simulink model "EkalmanF_ac_sim"  (R2025b)
settings: Solver=VariableStepAuto  StartTime=0.0  StopTime=StopTime  RelTol=1e-3
values from neighbouring files (symbols this model uses):
  B = [0.5*dt^2 0 ... (first row only)    [Extended_Kalman_Filter.m]    (also in Kalman_filter.m; kalman_ac.m = fi(B, true, 32, 20))
  C = fi(C, true, 32, 20)    [kalman_ac.m]
  dt = 0.2    [Extended_Kalman_Filter.m]    (also in Kalman_filter.m; UKF.m; kalman_ac.m = 0.02)
  H = [1 0 0 0 ... (first row only)    [Extended_Kalman_Filter.m]    (also in Kalman_filter.m; UKF.m; kalman_ac.m = fi(H, true, 32, 20))
  Q = 0.01 * eye(4)    [Extended_Kalman_Filter.m]    (also in Kalman_filter.m; UKF.m; kalman_ac.m = fi(Q, true, 32, 20))
  time = (1:num_steps) * dt    [Extended_Kalman_Filter.m]    (also in Kalman_filter.m; UKF.m; kalman_ac.m = single(0:dt:StopTime))
undefined symbols (not defined in the file or in its folder): T1, T10, T11, T12, T13, T14, T15, T16, T2, T3, T4, T5, T6, T7, T8, T9
libraries: dspsrcs4 x3, hdlsllib x3
settings Model: Creator=stefa  LastModifiedBy=Radu Editoriu
settings OptimizationCC: BlockReduction=off  ConditionallyExecuteInputs=off

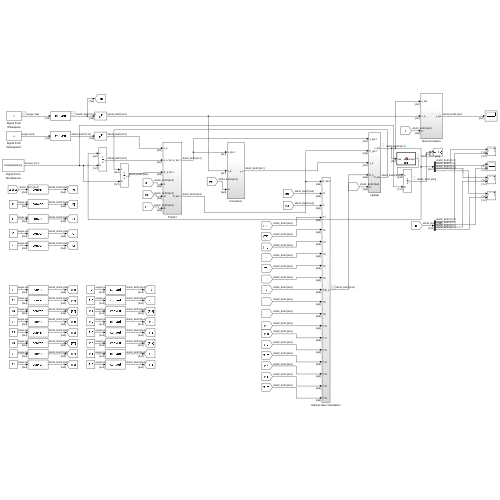
[thumbnail: Simulink's stored preview of the top-level diagram]
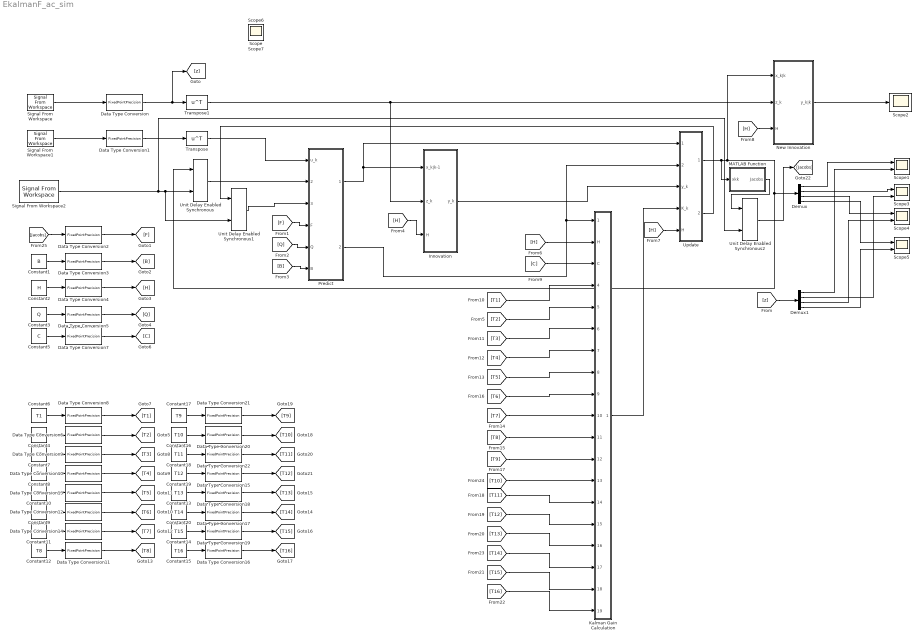
== system EkalmanF_ac_sim ==
  Constant1 : Constant  Value=B
  Constant10 : Constant  Value=T5
  Constant11 : Constant  Value=T7
  Constant12 : Constant  Value=T8
  Constant13 : Constant  Value=T13
  Constant14 : Constant  Value=T15
  Constant15 : Constant  Value=T16
  Constant16 : Constant  Value=T10
  Constant17 : Constant  Value=T9
  Constant18 : Constant  Value=T11
  Constant19 : Constant  Value=T12
  Constant2 : Constant  Value=H
  Constant20 : Constant  Value=T14
  Constant3 : Constant  Value=Q
  Constant4 : Constant  Value=T2
  Constant5 : Constant  Value=C
  Constant6 : Constant  Value=T1
  Constant7 : Constant  Value=T3
  Constant8 : Constant  Value=T4
  Constant9 : Constant  Value=T6
  Data Type Conversion : DataTypeConversion  OutMin=[1e-3]  OutMax=[1000]  OutDataTypeStr=FixedPointPrecision  SaturateOnIntegerOverflow=off  RndMeth=Floor
  Data Type Conversion{1..22} (22 alike) : DataTypeConversion  OutDataTypeStr=FixedPointPrecision  SaturateOnIntegerOverflow=off  RndMeth=Floor
  Demux : Demux
  Demux1 : Demux
  Innovation : Subsystem
  Kalman Gain Calculation : Subsystem
  MATLAB Function : MATLAB Function  TreatAsAtomicUnit=on
  New Innovation : Subsystem
  Predict : Subsystem
  Scope{1,3..5} (4 alike) : Scope  NumInputPorts=2
      Scope1 settings: ActiveDisplayYMinimum=0.82247254545106063  ActiveDisplayYMaximum=3.0989073933185614  DataLoggingSaveFormat=Array
      Scope3 settings: ActiveDisplayYMinimum=-1.2492327051740526  ActiveDisplayYMaximum=3.1864617109082456  DataLoggingVariableName=ScopeData2  DataLoggingSaveFormat=Array
      Scope4 settings: ActiveDisplayYMinimum=-5.84392599463885  ActiveDisplayYMaximum=2.7669674927194179  DataLoggingVariableName=ScopeData3  DataLoggingSaveFormat=Array
      Scope5 settings: ActiveDisplayYMinimum=-5.0260366041316269  ActiveDisplayYMaximum=3.5090934704886196  DataLoggingVariableName=ScopeData4  DataLoggingSaveFormat=Array
  Scope{,2,6..7} (4 alike) : Scope
      Scope2 settings: ActiveDisplayYMinimum=-1.1122805343511448  ActiveDisplayYMaximum=1.0927194656488552  DataLoggingSaveFormat=Array
      Scope settings: ActiveDisplayYMinimum=-9.1353842219735029  ActiveDisplayYMaximum=57.624373102579447  DataLoggingVariableName=ScopeData5
      Scope6 settings: ActiveDisplayYMinimum=-1  ActiveDisplayYMaximum=1  DataLoggingVariableName=ScopeData6
      Scope7 settings: ActiveDisplayYMinimum=-0.035523056983947747  ActiveDisplayYMaximum=0.31970751285552979  DataLoggingVariableName=ScopeData7
  Signal From Workspace : dspsrcs4/Signal From Workspace  X=z  Ts=dt  nsamps=1  OutputAfterFinalValue=Setting to zero  ignoreOrWarnInputAndFrameLengths=off  OutputFrames=off
  Signal From Workspace1 : dspsrcs4/Signal From Workspace  X=u  Ts=dt  nsamps=1  OutputAfterFinalValue=Setting to zero  ignoreOrWarnInputAndFrameLengths=off  OutputFrames=off
  Signal From Workspace2 : dspsrcs4/Signal From Workspace  X=true(size(time))  Ts=dt  nsamps=1  OutputAfterFinalValue=Setting to zero  ignoreOrWarnInputAndFrameLengths=off  OutputFrames=off
  Transpose : Math  Operator=transpose  SignedPower=on  RndMeth=Zero
  Transpose1 : Math  Operator=transpose  SignedPower=on  RndMeth=Zero
  Unit Delay Enabled Synchronous : hdlsllib/Discrete/Unit Delay Enabled Synchronous  InitialCondition=0.0  SampleTime=-1
  Unit Delay Enabled Synchronous1 : hdlsllib/Discrete/Unit Delay Enabled Synchronous  InitialCondition=0.0  SampleTime=-1
  Unit Delay Enabled Synchronous2 : hdlsllib/Discrete/Unit Delay Enabled Synchronous  InitialCondition=0.0  SampleTime=-1
  Update : Subsystem
  wires:
  Signal From Workspace1/1 -> Data Type Conversion1/1
  Signal From Workspace/1 -> Data Type Conversion/1
  Predict/1(x_k|k-1) -> Update/1(x_k|k-1), Innovation/1(x_k|k-1)
  Kalman Gain Calculation/1(K_k) -> Update/4(K_k)
  Innovation/1(y_k) -> Update/3(y_k)
  Update/1(x_k|k) -> MATLAB Function/1(xkk), New Innovation/1(x_k|k), Demux/1, Unit Delay Enabled Synchronous/1
  Update/2(P_k|k) -> Unit Delay Enabled Synchronous1/1
  Predict/2(P_k|k-1) -> Update/2(P_k|k-1), Kalman Gain Calculation/1(P_k|k-1)
  Unit Delay Enabled Synchronous/1 -> Predict/2(x_k-1|k-1)
  Unit Delay Enabled Synchronous1/1 -> Predict/3(P_k-1|k-1)
  Transpose/1 -> Predict/1(u_k)
  New Innovation/1(y_k|k) -> Scope2/1
  Demux/1 -> Scope1/1
  Demux/2 -> Scope3/1
  Demux/3 -> Scope4/1
  Demux/4 -> Scope5/1
  Transpose1/1 -> Innovation/2(z_k), New Innovation/2(z_k)
  [z] -> Demux1/1
  Demux1/1 -> Scope1/2
  Demux1/2 -> Scope3/2
  Demux1/3 -> Scope4/2
  Demux1/4 -> Scope5/2
  Data Type Conversion/1 -> [z], Transpose1/1
  Data Type Conversion1/1 -> Transpose/1
  Signal From Workspace2/1 -> Unit Delay Enabled Synchronous2/2, Unit Delay Enabled Synchronous/2, Unit Delay Enabled Synchronous1/2
  Data Type Conversion2/1 -> [F]
  Data Type Conversion3/1 -> [B]
  Data Type Conversion4/1 -> [H]
  Data Type Conversion5/1 -> [Q]
  Constant1/1 -> Data Type Conversion3/1
  Constant2/1 -> Data Type Conversion4/1
  Constant3/1 -> Data Type Conversion5/1
  [F] -> Predict/4(F)
  [Q] -> Predict/5(Q)
  [B] -> Predict/6(B)
  [H] -> Innovation/3(H)
  [H] -> Kalman Gain Calculation/2(H)
  [H] -> Update/5(H)
  [H] -> New Innovation/3(H)
  Constant5/1 -> Data Type Conversion7/1
  Data Type Conversion7/1 -> [C]
  Constant6/1 -> Data Type Conversion8/1
  Data Type Conversion8/1 -> [T1]
  [C] -> Kalman Gain Calculation/3(C)
  [T1] -> Kalman Gain Calculation/4(T1)
  Constant4/1 -> Data Type Conversion6/1
  Data Type Conversion6/1 -> [T2]
  Data Type Conversion9/1 -> [T3]
  Constant7/1 -> Data Type Conversion9/1
  Constant8/1 -> Data Type Conversion10/1
  Data Type Conversion10/1 -> [T4]
  Data Type Conversion12/1 -> [T6]
  Data Type Conversion11/1 -> [T8]
  Constant12/1 -> Data Type Conversion11/1
  Data Type Conversion14/1 -> [T7]
  Constant10/1 -> Data Type Conversion13/1
  Constant11/1 -> Data Type Conversion14/1
  Data Type Conversion13/1 -> [T5]
  Constant9/1 -> Data Type Conversion12/1
  Constant20/1 -> Data Type Conversion17/1
  Data Type Conversion19/1 -> [T15]
  Constant14/1 -> Data Type Conversion19/1
  Constant13/1 -> Data Type Conversion18/1
  Data Type Conversion16/1 -> [T16]
  Data Type Conversion17/1 -> [T14]
  Data Type Conversion18/1 -> [T13]
  Constant15/1 -> Data Type Conversion16/1
  Data Type Conversion20/1 -> [T10]
  Data Type Conversion15/1 -> [T12]
  Constant19/1 -> Data Type Conversion15/1
  Data Type Conversion22/1 -> [T11]
  Constant17/1 -> Data Type Conversion21/1
  Constant18/1 -> Data Type Conversion22/1
  Data Type Conversion21/1 -> [T9]
  Constant16/1 -> Data Type Conversion20/1
  [T2] -> Kalman Gain Calculation/5(T2)
  [T3] -> Kalman Gain Calculation/6(T3)
  [T4] -> Kalman Gain Calculation/7(T4)
  [T5] -> Kalman Gain Calculation/8(T5)
  [T6] -> Kalman Gain Calculation/9(T6)
  [T7] -> Kalman Gain Calculation/10(T7)
  [T8] -> Kalman Gain Calculation/11(T8)
  [T9] -> Kalman Gain Calculation/12(T9)
  [T10] -> Kalman Gain Calculation/13(T10)
  [T11] -> Kalman Gain Calculation/14(T11)
  [T12] -> Kalman Gain Calculation/15(T12)
  [T13] -> Kalman Gain Calculation/16(T13)
  [T14] -> Kalman Gain Calculation/17(T14)
  [T15] -> Kalman Gain Calculation/18(T15)
  [T16] -> Kalman Gain Calculation/19(T16)
  [Jacobs] -> Data Type Conversion2/1
  MATLAB Function/1(Jacobs) -> Unit Delay Enabled Synchronous2/1
  Unit Delay Enabled Synchronous2/1 -> [Jacobs]

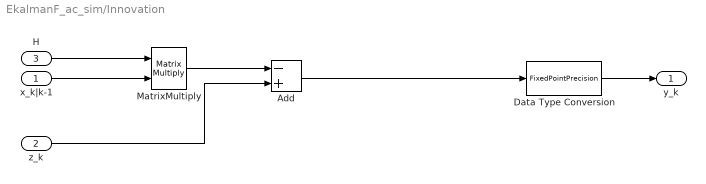
== system EkalmanF_ac_sim/Innovation ==
  x_k|k-1 : Inport
  z_k : Inport  Port=2
  H : Inport  Port=3
  Add : Sum  Inputs=-+
  Data Type Conversion : DataTypeConversion  OutDataTypeStr=FixedPointPrecision  SaturateOnIntegerOverflow=off  RndMeth=Floor
  MatrixMultiply : Product  Multiplication=Matrix(*)
  y_k : Outport
  wires:
  x_k|k-1/1 -> MatrixMultiply/2
  MatrixMultiply/1 -> Add/1
  z_k/1 -> Add/2
  Add/1 -> Data Type Conversion/1
  H/1 -> MatrixMultiply/1
  Data Type Conversion/1 -> y_k/1

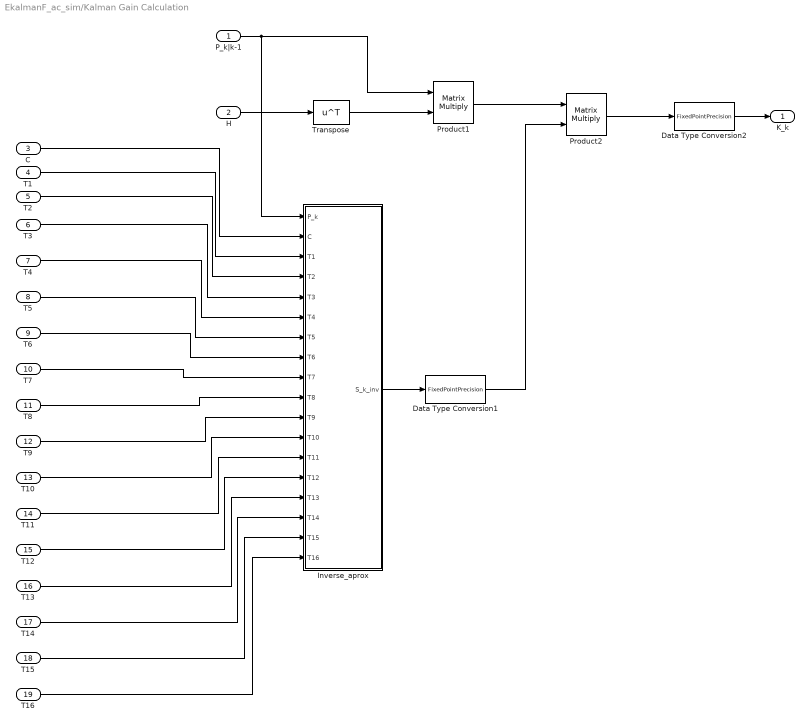
== system EkalmanF_ac_sim/Kalman Gain Calculation ==
  P_k|k-1 : Inport
  H : Inport  Port=2
  C : Inport  Port=3
  T1 : Inport  Port=4
  T2 : Inport  Port=5
  T3 : Inport  Port=6
  T4 : Inport  Port=7
  T5 : Inport  Port=8
  T6 : Inport  Port=9
  T7 : Inport  Port=10
  T8 : Inport  Port=11
  T9 : Inport  Port=12
  T10 : Inport  Port=13
  T11 : Inport  Port=14
  T12 : Inport  Port=15
  T13 : Inport  Port=16
  T14 : Inport  Port=17
  T15 : Inport  Port=18
  T16 : Inport  Port=19
  Data Type Conversion1 : DataTypeConversion  OutDataTypeStr=FixedPointPrecision  SaturateOnIntegerOverflow=off  RndMeth=Floor
  Data Type Conversion2 : DataTypeConversion  OutDataTypeStr=FixedPointPrecision  SaturateOnIntegerOverflow=off  RndMeth=Floor
  Inverse_aprox : MATLAB Function  TreatAsAtomicUnit=on
  Product1 : Product  Multiplication=Matrix(*)
  Product2 : Product  Multiplication=Matrix(*)
  Transpose : Math  Operator=transpose  SignedPower=on  RndMeth=Zero
  K_k : Outport
  wires:
  H/1 -> Transpose/1
  P_k|k-1/1 -> Product1/1, Inverse_aprox/1(P_k)
  Transpose/1 -> Product1/2
  Inverse_aprox/1(S_k_inv) -> Data Type Conversion1/1
  Product2/1 -> Data Type Conversion2/1
  Product1/1 -> Product2/1
  Data Type Conversion1/1 -> Product2/2
  Data Type Conversion2/1 -> K_k/1
  C/1 -> Inverse_aprox/2(C)
  T1/1 -> Inverse_aprox/3(T1)
  T2/1 -> Inverse_aprox/4(T2)
  T3/1 -> Inverse_aprox/5(T3)
  T4/1 -> Inverse_aprox/6(T4)
  T5/1 -> Inverse_aprox/7(T5)
  T6/1 -> Inverse_aprox/8(T6)
  T7/1 -> Inverse_aprox/9(T7)
  T8/1 -> Inverse_aprox/10(T8)
  T9/1 -> Inverse_aprox/11(T9)
  T10/1 -> Inverse_aprox/12(T10)
  T11/1 -> Inverse_aprox/13(T11)
  T12/1 -> Inverse_aprox/14(T12)
  T13/1 -> Inverse_aprox/15(T13)
  T14/1 -> Inverse_aprox/16(T14)
  T15/1 -> Inverse_aprox/17(T15)
  T16/1 -> Inverse_aprox/18(T16)

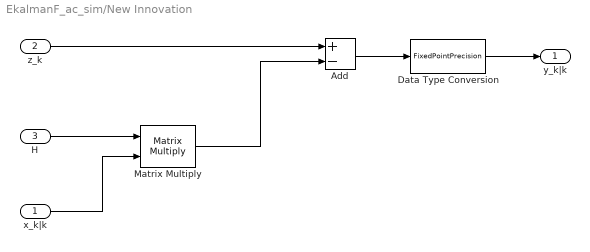
== system EkalmanF_ac_sim/New Innovation ==
  x_k|k : Inport
  z_k : Inport  Port=2
  H : Inport  Port=3
  Add : Sum  Inputs=+-
  Data Type Conversion : DataTypeConversion  OutDataTypeStr=FixedPointPrecision  SaturateOnIntegerOverflow=off  RndMeth=Floor
  Matrix Multiply : Product  Multiplication=Matrix(*)
  y_k|k : Outport
  wires:
  z_k/1 -> Add/1
  H/1 -> Matrix Multiply/1
  x_k|k/1 -> Matrix Multiply/2
  Matrix Multiply/1 -> Add/2
  Add/1 -> Data Type Conversion/1
  Data Type Conversion/1 -> y_k|k/1

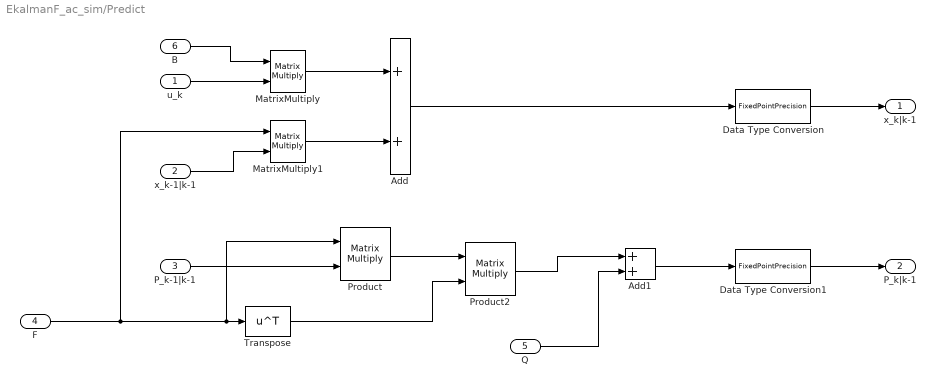
== system EkalmanF_ac_sim/Predict ==
  u_k : Inport
  x_k-1|k-1 : Inport  Port=2
  P_k-1|k-1 : Inport  Port=3
  F : Inport  Port=4
  Q : Inport  Port=5
  B : Inport  Port=6
  Add : Sum
  Add1 : Sum
  Data Type Conversion : DataTypeConversion  OutDataTypeStr=FixedPointPrecision  SaturateOnIntegerOverflow=off  RndMeth=Floor
  Data Type Conversion1 : DataTypeConversion  OutDataTypeStr=FixedPointPrecision  SaturateOnIntegerOverflow=off  RndMeth=Floor
  MatrixMultiply : Product  Multiplication=Matrix(*)
  MatrixMultiply1 : Product  Multiplication=Matrix(*)
  Product : Product  Multiplication=Matrix(*)
  Product2 : Product  Multiplication=Matrix(*)
  Transpose : Math  Operator=transpose  SignedPower=on  RndMeth=Zero
  x_k|k-1 : Outport
  P_k|k-1 : Outport  Port=2
  wires:
  x_k-1|k-1/1 -> MatrixMultiply1/2
  Add/1 -> Data Type Conversion/1
  MatrixMultiply1/1 -> Add/2
  MatrixMultiply/1 -> Add/1
  P_k-1|k-1/1 -> Product/2
  Q/1 -> Add1/2
  Add1/1 -> Data Type Conversion1/1
  Product2/1 -> Add1/1
  Product/1 -> Product2/1
  Transpose/1 -> Product2/2
  B/1 -> MatrixMultiply/1
  F/1 -> MatrixMultiply1/1, Transpose/1, Product/1
  Data Type Conversion/1 -> x_k|k-1/1
  Data Type Conversion1/1 -> P_k|k-1/1
  u_k/1 -> MatrixMultiply/2

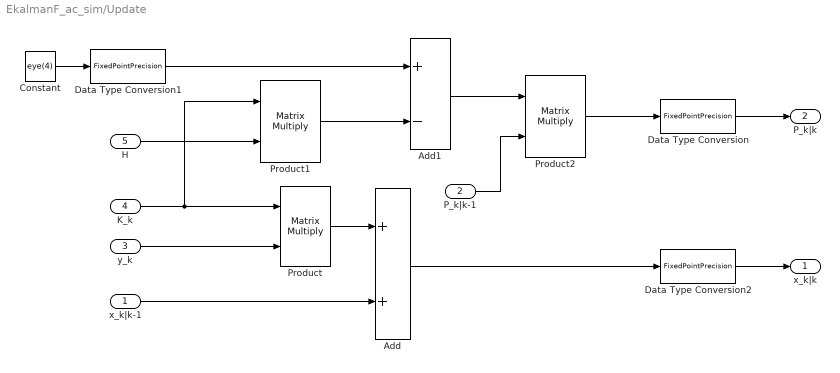
== system EkalmanF_ac_sim/Update ==
  x_k|k-1 : Inport
  P_k|k-1 : Inport  Port=2
  y_k : Inport  Port=3
  K_k : Inport  Port=4
  H : Inport  Port=5
  Add : Sum
  Add1 : Sum  Inputs=+-
  Constant : Constant  Value=eye(4)
  Data Type Conversion : DataTypeConversion  OutDataTypeStr=FixedPointPrecision  SaturateOnIntegerOverflow=off  RndMeth=Floor
  Data Type Conversion1 : DataTypeConversion  OutDataTypeStr=FixedPointPrecision  SaturateOnIntegerOverflow=off  RndMeth=Floor
  Data Type Conversion2 : DataTypeConversion  OutDataTypeStr=FixedPointPrecision  SaturateOnIntegerOverflow=off  RndMeth=Floor
  Product : Product  Multiplication=Matrix(*)
  Product1 : Product  Multiplication=Matrix(*)
  Product2 : Product  Multiplication=Matrix(*)
  x_k|k : Outport
  P_k|k : Outport  Port=2
  wires:
  K_k/1 -> Product1/1, Product/1
  y_k/1 -> Product/2
  Product/1 -> Add/1
  x_k|k-1/1 -> Add/2
  Add/1 -> Data Type Conversion2/1
  H/1 -> Product1/2
  Product1/1 -> Add1/2
  Constant/1 -> Data Type Conversion1/1
  P_k|k-1/1 -> Product2/2
  Add1/1 -> Product2/1
  Product2/1 -> Data Type Conversion/1
  Data Type Conversion1/1 -> Add1/1
  Data Type Conversion/1 -> P_k|k/1
  Data Type Conversion2/1 -> x_k|k/1

== matlab function EkalmanF_ac_sim/MATLAB Function ==
  data: xkk input; Jacobs output
function Jacobs = fcn(xkk)
%#codegen

Jacobs = [1 + 0.3*cos(xkk(1)), 0, 0.02, 0;
          0, 1 + 0.3*cos(xkk(2)), 0, 0.02;
          0, 0, 1, 0;
          0, 0, 0, 1];
end

== matlab function EkalmanF_ac_sim/Kalman Gain Calculation/Inverse_aprox ==
  data: S_k_inv output; P_k input; C input; T1 input; T2 input; T3 input; T4 input; T5 input; T6 input; T7 input; T8 input; T9 input; T10 input; T11 input; T12 input; T13 input; T14 input; T15 input; T16 input
function S_k_inv = inverse_aprox(P_k, C, T1, T2, T3, T4, T5, T6, T7, T8, T9, T10, T11, T12, T13, T14, T15, T16)
    Z = P_k - fi(eye(4),true, 66, 40);
    sum = fi(zeros(4,4),true, 66, 40);
    sum = sum + T1*Z(1,1);
    sum = sum + T2*Z(1,2);
    sum = sum + T3*Z(1,3);
    sum = sum + T4*Z(1,4);
    sum = sum + T5*Z(2,1);
    sum = sum + T6*Z(2,2);
    sum = sum + T7*Z(2,3);
    sum = sum + T8*Z(2,4);
    sum = sum + T9*Z(3,1);
    sum = sum + T10*Z(3,2);
    sum = sum + T11*Z(3,3);
    sum = sum + T12*Z(3,4);
    sum = sum + T13*Z(4,1);
    sum = sum + T14*Z(4,2);
    sum = sum + T15*Z(4,3);
    sum = sum + T16*Z(4,4);    
    S_k_inv = C - fi(sum, true, 32, 20);
end
